simulink model "ReferenceGeneratorxLQRCombinedxPWMGenerator"  (R2025b)
settings: Solver=FixedStepDiscrete  StartTime=0.0  StopTime=inf  FixedStep=0.005  RelTol=1e-3
settings Model: Creator=mwali  LastModifiedBy=hassa
settings OptimizationCC: DefaultParameterBehavior=Inlined  UseDivisionForNetSlopeComputation=on  GainParamInheritBuiltInType=on  UseFloatMulNetSlope=on  InlineInvariantSignals=on  PassReuseOutputArgsAs=Individual arguments  ZeroExternalMemoryAtStartup=off  ZeroInternalMemoryAtStartup=off  NoFixptDivByZeroProtection=on  EfficientFloat2IntCast=on  LifeSpan=1  MaxStackSize=512  OptimizeBlockOrder=speed  DifferentSizesBufferReuse=on  EfficientTunableParamExpr=on
settings DebuggingCC: ParameterTunabilityLossMsg=error
settings HardwareCC: ProdBitPerPointer=32.0  ProdBitPerSizeT=32.0  ProdBitPerPtrDiffT=32.0  ProdLargestAtomicInteger=Long  ProdLargestAtomicFloat=Double  ProdWordSize=32.0  ProdLongLongMode=on  ProdHWDeviceType=ARM Compatible->ARM Cortex-M
settings SFSimCC: MATLABDynamicMemAlloc=off
settings RTWCC: SystemTargetFile=ert.tlc  HardwareBoard=STM32H7xx Based (Single-core)  TemplateMakefile=ert_default_tmf  Toolchain=GNU Tools for ARM Embedded Processors  Description=Embedded Coder
settings CodeAppCC: ForceParamTrailComments=on  IgnoreCustomStorageClasses=off  OperatorAnnotations=on  SimulinkDataObjDesc=on  SFDataObjDesc=on  CustomSymbolStrGlobalVar=rt$N$M  CustomSymbolStrType=$N$M  CustomSymbolStrFcn=$N$M$F  CustomSymbolStrMacro=$N$M  InsertBlockDesc=on
settings ERTTargetCC: ExtModeTransport=3.0  ExtModeStaticAlloc=on  ExtModeStaticAllocSize=2048.0  ExtModeMexFile=ext_xcp  ExtModeIntrfLevel=Level2 - Open  ERTFilePackagingFormat=CompactWithDataFile  TargetLangStandard=C99 (ISO)  CodeReplacementLibrary=ARM Cortex-M  IncludeMdlTerminateFcn=off  CombineSignalStateStructs=on  SupportAbsoluteTime=off  SupportComplex=off  SupportNonInlinedSFcns=on

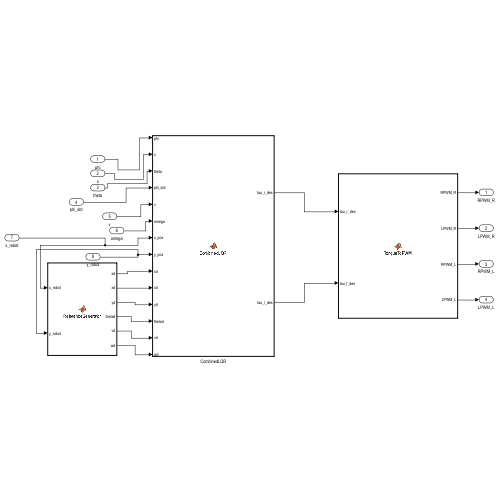
[thumbnail: Simulink's stored preview of the top-level diagram]
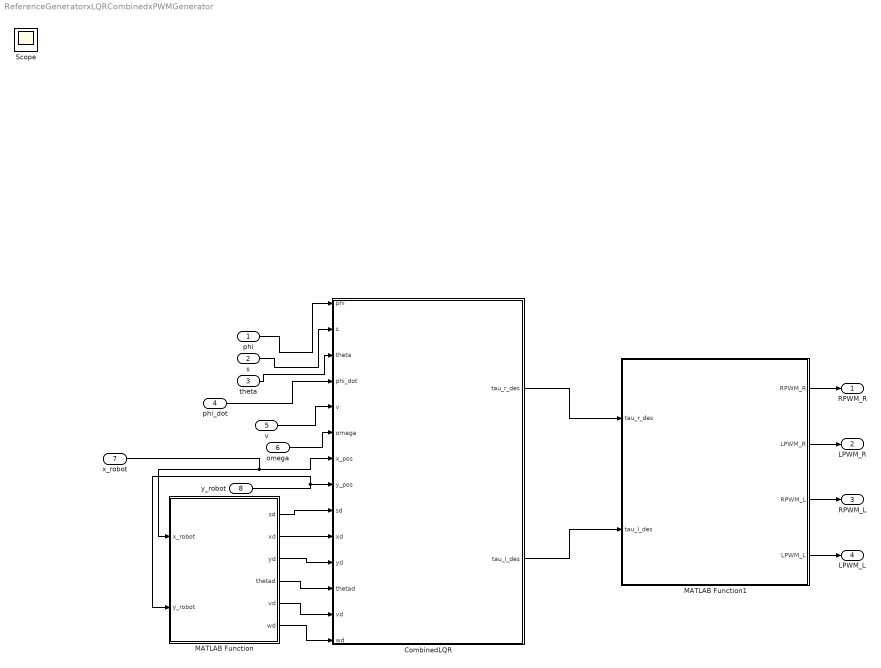
== system ReferenceGeneratorxLQRCombinedxPWMGenerator ==
  phi : Inport
  s : Inport  Port=2
  theta : Inport  Port=3
  phi_dot : Inport  Port=4
  v : Inport  Port=5
  omega : Inport  Port=6
  x_robot : Inport  Port=7
  y_robot : Inport  Port=8
  CombinedLQR : MATLAB Function  TreatAsAtomicUnit=on
  MATLAB Function : MATLAB Function  TreatAsAtomicUnit=on
  MATLAB Function1 : MATLAB Function  TreatAsAtomicUnit=on
  RPWM_R : Outport
  LPWM_R : Outport  Port=2
  RPWM_L : Outport  Port=3
  LPWM_L : Outport  Port=4
  Scope : Scope
      settings: ActiveDisplayYMinimum=-0.34848844243079913  ActiveDisplayYMaximum=2.6945477005962535
  wires:
  MATLAB Function/2(xd) -> CombinedLQR/10(xd)
  phi_dot/1 -> CombinedLQR/4(phi_dot)
  theta/1 -> CombinedLQR/3(theta)
  MATLAB Function/3(yd) -> CombinedLQR/11(yd)
  y_robot/1 -> MATLAB Function/2(y_robot), CombinedLQR/8(y_pos)
  v/1 -> CombinedLQR/5(v)
  omega/1 -> CombinedLQR/6(omega)
  x_robot/1 -> CombinedLQR/7(x_pos), MATLAB Function/1(x_robot)
  s/1 -> CombinedLQR/2(s)
  MATLAB Function1/2(LPWM_R) -> LPWM_R/1
  MATLAB Function1/1(RPWM_R) -> RPWM_R/1
  MATLAB Function/1(sd) -> CombinedLQR/9(sd)
  CombinedLQR/1(tau_r_des) -> MATLAB Function1/1(tau_r_des)
  CombinedLQR/2(tau_l_des) -> MATLAB Function1/2(tau_l_des)
  MATLAB Function/6(wd) -> CombinedLQR/14(wd)
  MATLAB Function/4(thetad) -> CombinedLQR/12(thetad)
  phi/1 -> CombinedLQR/1(phi)
  MATLAB Function/5(vd) -> CombinedLQR/13(vd)
  MATLAB Function1/3(RPWM_L) -> RPWM_L/1
  MATLAB Function1/4(LPWM_L) -> LPWM_L/1

== matlab function ReferenceGeneratorxLQRCombinedxPWMGenerator/CombinedLQR ==
  settings: updateMethod=DISCRETE
  data: phi input; s input; theta input; phi_dot input; v input; omega input; x_pos input; y_pos input; sd input; xd input; yd input; thetad input; vd input; wd input; tau_r_des output; tau_l_des output
function [tau_r_des, tau_l_des] = CombinedLQR( ...
    phi, s, theta, phi_dot, v, omega, x_pos, y_pos, ...
    sd, xd, yd, thetad, vd, wd)
%#codegen

% LQR Gain Matrix
K_lqr = [-16.616882069954595	-1.118033988749899	3.162277660168384	-2.938330914554923	-2.061355185548641	1.622468529505869;
-16.616882069954599	-1.118033988749900	-3.162277660168376	-2.938330914554922	-2.061355185548644	-1.622468529505866];

% outputs init
tau_r_des  = 0;
tau_l_des  = 0;
ex_out     = 0;
ey_out     = 0;
etheta_out = 0;

% -----------------------------
% STATIC EQUILIBRIUM CONSTANT
% -----------------------------
% Based on Low Posture (Lc = 170.9 mm, X-COM shift = 0.56 mm)
X_com_offset = 0.00056; 
Lc = 0.1709;
phi_ref = atan(X_com_offset / Lc); 

% -----------------------------
% 1) Path position error in world frame
% -----------------------------
dx = xd - x_pos;
dy = yd - y_pos;

% -----------------------------
% 2) Error in robot body frame
% -----------------------------
ex =  cos(theta)*dx + sin(theta)*dy;
ey = -sin(theta)*dx + cos(theta)*dy;

% save for plotting
ex_out = ex;
ey_out = ey;

% -----------------------------
% 3) Heading correction from lateral error
% -----------------------------
k_y = 0.1;                     % tune this if needed
theta_corr_max = deg2rad(20);  % max heading correction

theta_corr = k_y * ey;

if theta_corr > theta_corr_max
    theta_corr = theta_corr_max;
elseif theta_corr < -theta_corr_max
    theta_corr = -theta_corr_max;
end

thetad_corr = thetad + theta_corr;

% -----------------------------
% 4) State error for LQR
% -----------------------------
e = zeros(6,1);

% Error is now actual tilt minus the static equilibrium constant
e(1) = phi - phi_ref; 
e(2) = s - sd; 
e(3) = atan2(sin(theta - thetad_corr), cos(theta - thetad_corr));
e(4) = phi_dot;
e(5) = v - vd;
e(6) = omega - wd;

etheta_out = e(3);

% -----------------------------
% 5) LQR control
% -----------------------------
u_des = -K_lqr * e;

tau_r_des = u_des(1);
tau_l_des = u_des(2);

% -----------------------------
% 6) Torque saturation
% -----------------------------
tau_lim = 3; 

if tau_r_des > tau_lim
    tau_r_des = tau_lim;
elseif tau_r_des < -tau_lim
    tau_r_des = -tau_lim;
end

if tau_l_des > tau_lim
    tau_l_des = tau_lim;
elseif tau_l_des < -tau_lim
    tau_l_des = -tau_lim;
end

== matlab function ReferenceGeneratorxLQRCombinedxPWMGenerator/MATLAB Function ==
  data: x_robot input; y_robot input; sd output; xd output; yd output; thetad output; vd output; wd output
function [sd, xd, yd, thetad, vd, wd] = ReferenceGenerator(x_robot, y_robot)
% --- PASTE THIS DIRECTLY INTO YOUR REFERENCE GENERATOR ---

S_path = [
    0.000000;
    0.454545;
    0.909091;
    1.363636;
    1.818182;
    2.272727;
    2.727273;
    3.181818;
    3.636364;
    4.090909;
    4.545455;
    5.000000;
    5.454545;
    5.909091;
    6.363636;
    6.818182;
    7.272727;
    7.727273;
    8.181818;
    8.636364;
    9.090909;
    9.545455;
    10.000000;
    10.454545;
    10.909091;
    11.363636;
    11.818182;
    12.272727;
    12.727273;
    13.181818;
    13.636364;
    14.090909;
    14.545455;
    15.000000;
    15.454545;
    15.909091;
    16.363636;
    16.818182;
    17.272727;
    17.727273;
    18.181818;
    18.636364;
    19.090909;
    19.545455;
    20.000000;
    20.454545;
    20.909091;
    21.363636;
    21.818182;
    22.272727;
    22.727273;
    23.181818;
    23.636364;
    24.090909;
    24.545455;
    25.000000;
    25.454545;
    25.909091;
    26.363636;
    26.818182;
    27.272727;
    27.727273;
    28.181818;
    28.636364;
    29.090909;
    29.545455;
    30.000000;
    30.454545;
    30.909091;
    31.363636;
    31.818182;
    32.272727;
    32.727273;
    33.181818;
    33.636364;
    34.090909;
    34.545455;
    35.000000;
    35.454545;
    35.909091;
    36.363636;
    36.818182;
    37.272727;
    37.727273;
    38.181818;
    38.636364;
    39.090909;
    39.545455;
    40.000000;
    40.454545;
    40.909091;
    41.363636;
    41.818182;
    42.272727;
    42.727273;
    43.181818;
    43.636364;
    44.090909;
    44.545455;
    45.000000;
];

P = [
    0.000000,  0.000000;
    0.454545,  0.000000;
    0.909091,  0.000000;
    1.363636,  0.000000;
    1.818182,  0.000000;
    2.272727,  0.000000;
    2.727273,  0.000000;
    3.181818,  0.000000;
    3.636364,  0.000000;
    4.090909,  0.000000;
    4.545455,  0.000000;
    5.000000,  0.000000;
    5.454545,  0.000000;
    5.909091,  0.000000;
    6.363636,  0.000000;
    6.818182,  0.000000;
    7.272727,  0.000000;
    7.727273,  0.000000;
    8.181818,  0.000000;
    8.636364,  0.000000;
    9.090909,  0.000000;
    9.545455,  0.000000;
    10.000000,  0.000000;
    10.454545,  0.000000;
    10.909091,  0.000000;
    11.363636,  0.000000;
    11.818182,  0.000000;
    12.272727,  0.000000;
    12.727273,  0.000000;
    13.181818,  0.000000;
    13.636364,  0.000000;
    14.090909,  0.000000;
    14.545455,  0.000000;
    15.000000,  0.000000;
    15.454545,  0.000000;
    15.909091,  0.000000;
    16.363636,  0.000000;
    16.818182,  0.000000;
    17.272727,  0.000000;
    17.727273,  0.000000;
    18.181818,  0.000000;
    18.636364,  0.000000;
    19.090909,  0.000000;
    19.545455,  0.000000;
    20.000000,  0.000000;
    20.454545,  0.000000;
    20.909091,  0.000000;
    21.363636,  0.000000;
    21.818182,  0.000000;
    22.272727,  0.000000;
    22.727273,  0.000000;
    23.181818,  0.000000;
    23.636364,  0.000000;
    24.090909,  0.000000;
    24.545455,  0.000000;
    25.000000,  0.000000;
    25.454545,  0.000000;
    25.909091,  0.000000;
    26.363636,  0.000000;
    26.818182,  0.000000;
    27.272727,  0.000000;
    27.727273,  0.000000;
    28.181818,  0.000000;
    28.636364,  0.000000;
    29.090909,  0.000000;
    29.545455,  0.000000;
    30.000000,  0.000000;
    30.454545,  0.000000;
    30.909091,  0.000000;
    31.363636,  0.000000;
    31.818182,  0.000000;
    32.272727,  0.000000;
    32.727273,  0.000000;
    33.181818,  0.000000;
    33.636364,  0.000000;
    34.090909,  0.000000;
    34.545455,  0.000000;
    35.000000,  0.000000;
    35.454545,  0.000000;
    35.909091,  0.000000;
    36.363636,  0.000000;
    36.818182,  0.000000;
    37.272727,  0.000000;
    37.727273,  0.000000;
    38.181818,  0.000000;
    38.636364,  0.000000;
    39.090909,  0.000000;
    39.545455,  0.000000;
    40.000000,  0.000000;
    40.454545,  0.000000;
    40.909091,  0.000000;
    41.363636,  0.000000;
    41.818182,  0.000000;
    42.272727,  0.000000;
    42.727273,  0.000000;
    43.181818,  0.000000;
    43.636364,  0.000000;
    44.090909,  0.000000;
    44.545455,  0.000000;
    45.000000,  0.000000;
];

theta_ref_unwrapped = [
    0.000000;
    0.000000;
    0.000000;
    0.000000;
    0.000000;
    0.000000;
    0.000000;
    0.000000;
    0.000000;
    0.000000;
    0.000000;
    0.000000;
    0.000000;
    0.000000;
    0.000000;
    0.000000;
    0.000000;
    0.000000;
    0.000000;
    0.000000;
    0.000000;
    0.000000;
    0.000000;
    0.000000;
    0.000000;
    0.000000;
    0.000000;
    0.000000;
    0.000000;
    0.000000;
    0.000000;
    0.000000;
    0.000000;
    0.000000;
    0.000000;
    0.000000;
    0.000000;
    0.000000;
    0.000000;
    0.000000;
    0.000000;
    0.000000;
    0.000000;
    0.000000;
    0.000000;
    0.000000;
    0.000000;
    0.000000;
    0.000000;
    0.000000;
    0.000000;
    0.000000;
    0.000000;
    0.000000;
    0.000000;
    0.000000;
    0.000000;
    0.000000;
    0.000000;
    0.000000;
    0.000000;
    0.000000;
    0.000000;
    0.000000;
    0.000000;
    0.000000;
    0.000000;
    0.000000;
    0.000000;
    0.000000;
    0.000000;
    0.000000;
    0.000000;
    0.000000;
    0.000000;
    0.000000;
    0.000000;
    0.000000;
    0.000000;
    0.000000;
    0.000000;
    0.000000;
    0.000000;
    0.000000;
    0.000000;
    0.000000;
    0.000000;
    0.000000;
    0.000000;
    0.000000;
    0.000000;
    0.000000;
    0.000000;
    0.000000;
    0.000000;
    0.000000;
    0.000000;
    0.000000;
    0.000000;
    0.000000;
];

vd_path = [
    1.000000;
    1.000000;
    1.000000;
    1.000000;
    1.000000;
    1.000000;
    1.000000;
    1.000000;
    1.000000;
    1.000000;
    1.000000;
    1.000000;
    1.000000;
    1.000000;
    1.000000;
    1.000000;
    1.000000;
    1.000000;
    1.000000;
    1.000000;
    1.000000;
    1.000000;
    1.000000;
    1.000000;
    1.000000;
    1.000000;
    1.000000;
    1.000000;
    1.000000;
    1.000000;
    1.000000;
    1.000000;
    1.000000;
    1.000000;
    1.000000;
    1.000000;
    1.000000;
    1.000000;
    1.000000;
    1.000000;
    1.000000;
    1.000000;
    1.000000;
    1.000000;
    1.000000;
    1.000000;
    1.000000;
    1.000000;
    1.000000;
    1.000000;
    1.000000;
    1.000000;
    1.000000;
    1.000000;
    1.000000;
    1.000000;
    1.000000;
    1.000000;
    1.000000;
    1.000000;
    1.000000;
    1.000000;
    1.000000;
    1.000000;
    1.000000;
    1.000000;
    1.000000;
    1.000000;
    1.000000;
    1.000000;
    1.000000;
    1.000000;
    1.000000;
    1.000000;
    1.000000;
    1.000000;
    1.000000;
    1.000000;
    1.000000;
    1.000000;
    1.000000;
    1.000000;
    1.000000;
    1.000000;
    1.000000;
    1.000000;
    1.000000;
    1.000000;
    1.000000;
    1.000000;
    1.000000;
    1.000000;
    1.000000;
    1.000000;
    1.000000;
    1.000000;
    1.000000;
    1.000000;
    1.000000;
    1.000000;
];

wd_path = [
    0.000000;
    0.000000;
    0.000000;
    0.000000;
    0.000000;
    0.000000;
    0.000000;
    0.000000;
    0.000000;
    0.000000;
    0.000000;
    0.000000;
    0.000000;
    0.000000;
    0.000000;
    0.000000;
    0.000000;
    0.000000;
    0.000000;
    0.000000;
    0.000000;
    0.000000;
    0.000000;
    0.000000;
    0.000000;
    0.000000;
    0.000000;
    0.000000;
    0.000000;
    0.000000;
    0.000000;
    0.000000;
    0.000000;
    0.000000;
    0.000000;
    0.000000;
    0.000000;
    0.000000;
    0.000000;
    0.000000;
    0.000000;
    0.000000;
    0.000000;
    0.000000;
    0.000000;
    0.000000;
    0.000000;
    0.000000;
    0.000000;
    0.000000;
    0.000000;
    0.000000;
    0.000000;
    0.000000;
    0.000000;
    0.000000;
    0.000000;
    0.000000;
    0.000000;
    0.000000;
    0.000000;
    0.000000;
    0.000000;
    0.000000;
    0.000000;
    0.000000;
    0.000000;
    0.000000;
    0.000000;
    0.000000;
    0.000000;
    0.000000;
    0.000000;
    0.000000;
    0.000000;
    0.000000;
    0.000000;
    0.000000;
    0.000000;
    0.000000;
    0.000000;
    0.000000;
    0.000000;
    0.000000;
    0.000000;
    0.000000;
    0.000000;
    0.000000;
    0.000000;
    0.000000;
    0.000000;
    0.000000;
    0.000000;
    0.000000;
    0.000000;
    0.000000;
    0.000000;
    0.000000;
    0.000000;
    0.000000;
];


    N = size(P, 1);

    % 1. Find the nearest discrete node
    min_dist2 = inf;
    k_min = int32(1);
    for k = int32(1) : int32(N)
        dx = P(k, 1) - x_robot;
        dy = P(k, 2) - y_robot;
        d2 = dx*dx + dy*dy;
        if d2 < min_dist2
            min_dist2 = d2;
            k_min = k;
        end
    end

    % 2. Continuous Projection (Fixes the high-frequency torque chattering)
    k_next = min(k_min + int32(1), int32(N));
    k_prev = max(k_min - int32(1), int32(1));

    d2_next = (P(k_next,1)-x_robot)^2 + (P(k_next,2)-y_robot)^2;
    d2_prev = (P(k_prev,1)-x_robot)^2 + (P(k_prev,2)-y_robot)^2;

    if d2_next < d2_prev
        k1 = k_min;
        k2 = k_next;
    else
        k1 = k_prev;
        k2 = k_min;
    end

    if k1 == k2
        alpha = 0.0;
    else
        vx = P(k2,1) - P(k1,1);
        vy = P(k2,2) - P(k1,2);
        L2 = vx*vx + vy*vy;
        if L2 > 1e-6
            rx = x_robot - P(k1,1);
            ry = y_robot - P(k1,2);
            % Orthogonal projection scalar
            alpha = (rx*vx + ry*vy) / L2;
            alpha = max(0.0, min(1.0, alpha));
        else
            alpha = 0.0;
        end
    end

    % 3. Interpolate perfectly smooth references (No Lookahead)
    sd     = (1 - alpha) * S_path(k1) + alpha * S_path(k2);
    xd     = (1 - alpha) * P(k1, 1)   + alpha * P(k2, 1);
    yd     = (1 - alpha) * P(k1, 2)   + alpha * P(k2, 2);
    thetad = (1 - alpha) * theta_ref_unwrapped(k1) + alpha * theta_ref_unwrapped(k2);
    vd     = (1 - alpha) * vd_path(k1) + alpha * vd_path(k2);
    wd     = (1 - alpha) * wd_path(k1) + alpha * wd_path(k2);

    % 4. Safety clamps
    vd_max = 0.3;
    wd_max = 0.334;
    vd = max(0, min(vd, vd_max));
    wd = max(min(wd, wd_max), -wd_max);
end

== matlab function ReferenceGeneratorxLQRCombinedxPWMGenerator/MATLAB Function1 ==
  data: tau_r_des input; RPWM_R output; tau_l_des input; LPWM_R output; RPWM_L output; LPWM_L output
function [RPWM_R, LPWM_R, RPWM_L, LPWM_L] = TorqueToPWM(tau_r_des, tau_l_des)
    % --- NFP-42GP-775-EN Motor Parameters ---
    Rated_Torque = 4.5;     
    DEADBAND_OFFSET = 130;
    
    % --- Controller & Robot Parameters ---
    max_pwm = 4000;    
    max_allowable_pwm = 3500;
    
    % Convert to base PWM
    pwm_r = round((tau_r_des / Rated_Torque) * max_pwm);
    pwm_l = round((tau_l_des / Rated_Torque) * max_pwm);
    
    % Apply deadband only if PWM is non-zero
    if pwm_r ~= 0
        pwm_r = pwm_r + (sign(pwm_r) * DEADBAND_OFFSET);
    end
    if pwm_l ~= 0
        pwm_l = pwm_l + (sign(pwm_l) * DEADBAND_OFFSET);
    end
    
    % Clamping logic
    pwm_r = max(min(pwm_r, max_allowable_pwm), -max_allowable_pwm);
    pwm_l = max(min(pwm_l, max_allowable_pwm), -max_allowable_pwm);
    
    % Directional H-Bridge splitting
    RPWM_R = max(0, pwm_r);
    LPWM_R = max(0, -pwm_r);
    
    RPWM_L = max(0, pwm_l);
    LPWM_L = max(0, -pwm_l);
end
